simulink model "opt_solver_2022"  (R2022a)
settings: Solver=FixedStepAuto  StartTime=0.0  StopTime=10.0  RelTol=1e-3
settings Model: Creator=SUN Runtong  LastModifiedBy=randolf
settings SolverCC: AlgebraicLoopSolver=TrustRegion
settings DataIOCC: ReturnWorkspaceOutputs=off
settings OptimizationCC: LocalBlockOutputs=off
settings DebuggingCC: UnconnectedInputMsg=warning  UnconnectedOutputMsg=warning  UnconnectedLineMsg=warning  SFMachineParentedDataDiag=warning  ArithmeticOperatorsInVariantConditions=warning
settings SFSimCC: CustomCodeUndefinedFunction=UseInterfaceOnly  SimTargetLang=C++
settings RTWCC: Description=TwinCAT Target  SystemTargetFile=TwinCAT.tlc  GenCodeOnly=on  MakeCommand=make_tct  TemplateMakefile=tct_msbuild.tmf  GenerateReport=on  TargetLang=C++
settings STFCustomTargetCC: TargetLangStandard=C++03 (ISO)  CompOptLevelCompliant=on  MATLABClassNameForMDSCustomization=Simulink.SoftwareTarget.TargetSpecificTriggerConfigurationBase  SystemTargetFile=TwinCAT.tlc

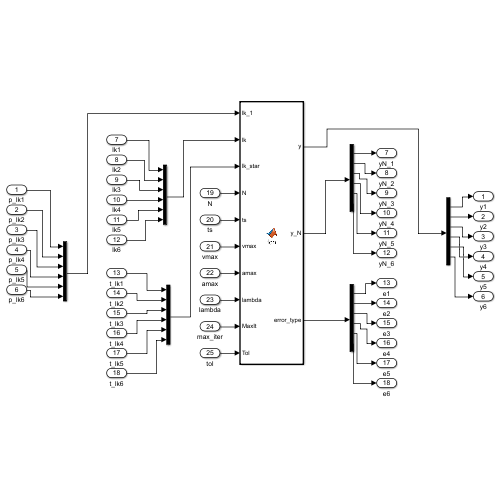
[thumbnail: Simulink's stored preview of the top-level diagram]
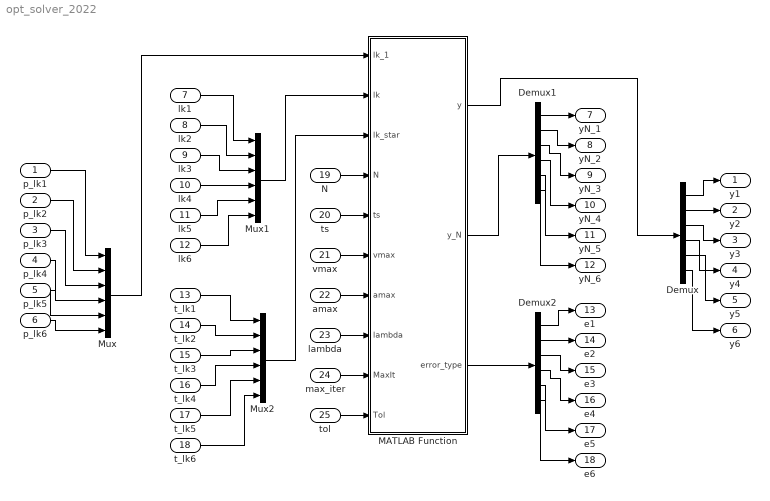
== system opt_solver_2022 ==
  p_lk1 : Inport
  p_lk2 : Inport  Port=2
  p_lk3 : Inport  Port=3
  p_lk4 : Inport  Port=4
  p_lk5 : Inport  Port=5
  p_lk6 : Inport  Port=6
  lk1 : Inport  Port=7
  lk2 : Inport  Port=8
  lk3 : Inport  Port=9
  lk4 : Inport  Port=10
  lk5 : Inport  Port=11
  lk6 : Inport  Port=12
  t_lk1 : Inport  Port=13
  t_lk2 : Inport  Port=14
  t_lk3 : Inport  Port=15
  t_lk4 : Inport  Port=16
  t_lk5 : Inport  Port=17
  t_lk6 : Inport  Port=18
  N : Inport  Port=19
  ts : Inport  Port=20
  vmax : Inport  Port=21
  amax : Inport  Port=22
  lambda : Inport  Port=23
  max_iter : Inport  Port=24
  tol : Inport  Port=25
  Demux : Demux  Outputs=6
  Demux1 : Demux  Outputs=6
  Demux2 : Demux  Outputs=6
  MATLAB Function : MATLAB Function  TreatAsAtomicUnit=on
  Mux : Mux  Inputs=6
  Mux1 : Mux  Inputs=6
  Mux2 : Mux  Inputs=6
  y1 : Outport
  y2 : Outport  Port=2
  y3 : Outport  Port=3
  y4 : Outport  Port=4
  y5 : Outport  Port=5
  y6 : Outport  Port=6
  yN_1 : Outport  Port=7
  yN_2 : Outport  Port=8
  yN_3 : Outport  Port=9
  yN_4 : Outport  Port=10
  yN_5 : Outport  Port=11
  yN_6 : Outport  Port=12
  e1 : Outport  Port=13
  e2 : Outport  Port=14
  e3 : Outport  Port=15
  e4 : Outport  Port=16
  e5 : Outport  Port=17
  e6 : Outport  Port=18
  wires:
  Demux/1 -> y1/1
  Demux/2 -> y2/1
  Demux/3 -> y3/1
  Demux/4 -> y4/1
  Demux/5 -> y5/1
  Demux/6 -> y6/1
  Demux1/3 -> yN_3/1
  Demux1/1 -> yN_1/1
  Demux1/2 -> yN_2/1
  Demux1/6 -> yN_6/1
  Demux1/5 -> yN_5/1
  Demux1/4 -> yN_4/1
  Demux2/3 -> e3/1
  Demux2/1 -> e1/1
  Demux2/2 -> e2/1
  Demux2/6 -> e6/1
  Demux2/5 -> e5/1
  Demux2/4 -> e4/1
  p_lk1/1 -> Mux/1
  p_lk2/1 -> Mux/2
  p_lk3/1 -> Mux/3
  p_lk4/1 -> Mux/4
  p_lk5/1 -> Mux/5
  p_lk6/1 -> Mux/6
  lk6/1 -> Mux1/6
  lk5/1 -> Mux1/5
  lk3/1 -> Mux1/3
  lk2/1 -> Mux1/2
  lk4/1 -> Mux1/4
  lk1/1 -> Mux1/1
  t_lk6/1 -> Mux2/6
  t_lk5/1 -> Mux2/5
  t_lk3/1 -> Mux2/3
  t_lk2/1 -> Mux2/2
  t_lk4/1 -> Mux2/4
  t_lk1/1 -> Mux2/1
  Mux/1 -> MATLAB Function/1(lk_1)
  N/1 -> MATLAB Function/4(N)
  ts/1 -> MATLAB Function/5(ts)
  vmax/1 -> MATLAB Function/6(vmax)
  amax/1 -> MATLAB Function/7(amax)
  lambda/1 -> MATLAB Function/8(lambda)
  max_iter/1 -> MATLAB Function/9(MaxIt)
  tol/1 -> MATLAB Function/10(Tol)
  MATLAB Function/1(y) -> Demux/1
  MATLAB Function/2(y_N) -> Demux1/1
  MATLAB Function/3(error_type) -> Demux2/1
  Mux1/1 -> MATLAB Function/2(lk)
  Mux2/1 -> MATLAB Function/3(lk_star)

== matlab function opt_solver_2022/MATLAB Function ==
  data: lk_1 input; y output; y_N output; lk input; lk_star input; N input; ts input; vmax input; amax input; lambda input; error_type output; MaxIt input; Tol input
function [y, y_N , error_type] = fcn(lk_1,lk,lk_star,N,ts,vmax,amax,lambda,MaxIt,Tol)
    y = zeros(6,1);
    y_N = zeros(6,1);
    error_type = zeros(6,1);
    %%构建对六个轴一样的矩阵
    H = diag([2*lambda*ones(1,N-1) 1+lambda]) - 2*lambda*diag([ones(N-1,1)],-1);
    H = 1/2*(H+H');
    Av = eye(N) - diag(ones(N-1,1),-1);
    Aa = eye(N) - 2*diag(ones(N-1,1),-1) + diag(ones(N-2,1),-2);
    A = [Av;
        -Av;
        Aa;
        -Aa];
    bv_base = ts*vmax*ones(2*N,1);
    bv = zeros(2*N,1);
    ba_base = ts^2*amax*ones(2*N,1);
    ba = zeros(2*N,1);
    %%%% to do: +向量维度判断
    
    for i = 1:6
        f = [-2*lambda*lk(i)
            zeros(N-2,1)
            -2*lk_star(i)];
        bv = bv_base;
        bv(1) = bv_base(1) + lk(i);
        bv(N+1) = bv_base(N+1) - lk(i); 
        ba = ba_base;
        ba(1) = ba_base(1) - lk_1(i) + 2*lk(i);
        ba(2) = ba_base(2) - lk(i);
        ba(N+1) = ba_base(N+1) + lk_1(i) - 2*lk(i);
        ba(N+2) = ba_base(N+2) + lk(i);
        b = [bv
            ba];
        [x,iter] = MyQP(2*H,f,A,b,[],[],lk(i)*ones(N,1),MaxIt,Tol);
        % if out of planning
        % 1=> true, prime number =>false
        % 2=> size error
        % 3=> null error
        % 5=> iter error
        % 7=> speed error
        % 11=> acc error
        error_type(i) = 1;
        % size error
        if (size(x,1)~=N)
            error_type(i) = error_type(i)*2;
        end
         % null error
        if (sum(isnan(x))>0)
            error_type(i) = error_type(i)*3;
        end
        % iteration
        if (iter>MaxIt)
            error_type(i) = error_type(i)*5;
        end
        % if speed out bound
        if (abs(x(1)-lk(i))>vmax*ts+1e-8)
           error_type(i) = error_type(i)*7; 
        end
        % if acceleration out bound
        if (abs(x(1)-2*lk(i)+lk_1(i))>amax*ts*ts+1e-8)
           error_type(i) = error_type(i)*11; 
        end
        
        if abs(error_type(i) - 1) < 1e-4
            y(i) = x(1);
            y_N(i) = x(N);
        else
            y(i) = lk(i);
        end
    end % end for i=1:6
end
